simulink model "DT4V_System_Model_v17_ref_speed_R2019a"  (R2023a)
settings: Solver=ode4  StartTime=0.0  StopTime=Config.Tsim  FixedStep=Config.Ts  RelTol=1e-3
undefined symbols (not defined in the file or in its folder): CC, Config, DCL, DiscIntNeverNeededParam, EM, GB, Grid, Inv, LM, Ma_1D, Psw_1D, Rceon_1D, Rec, Vceon_1D
libraries: simulink x3, DT4V_LoadModels x2
(part 1 of 2)
settings Model: TunableVars=Inv,Vceon_1D,Ma_1D,Psw_1D,Rceon_1D  TunableVarsStorageClass=Auto,Auto,Auto,Auto,Auto  TunableVarsTypeQualifier=,,,,  Creator=kjvthuyn  LastModifiedBy=megle
settings SolverCC: AlgebraicLoopSolver=TrustRegion
settings DebuggingCC: UnconnectedInputMsg=warning  UnconnectedOutputMsg=warning  UnconnectedLineMsg=warning
settings ModelReferenceCC: EnableRefExpFcnMdlSchedulingChecks=on
settings SFSimCC: CustomCodeUndefinedFunction=UseInterfaceOnly

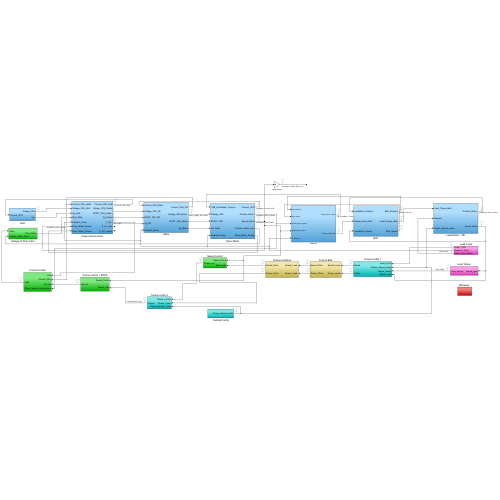
[thumbnail: Simulink's stored preview of the top-level diagram]
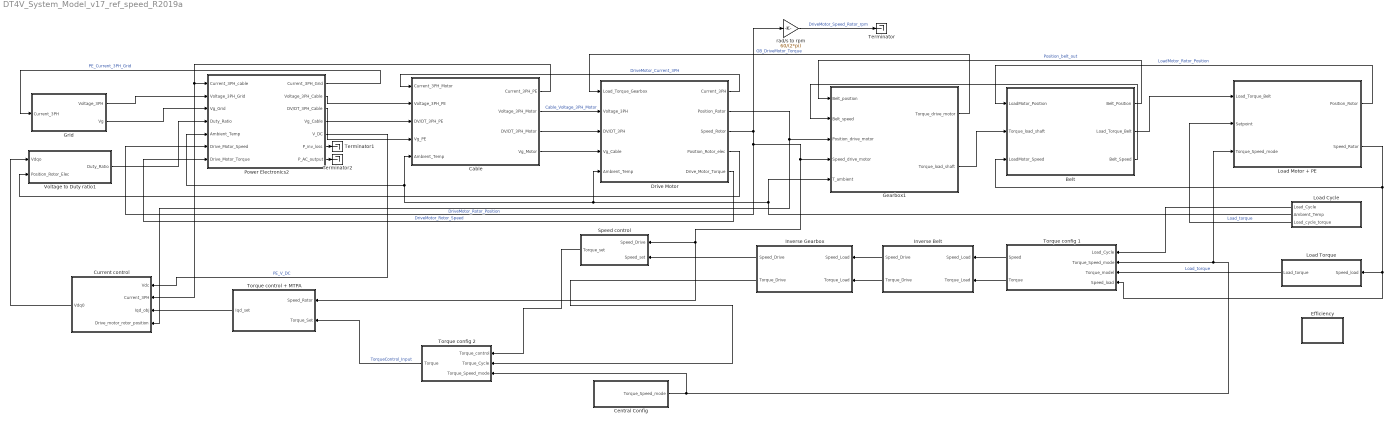
== system DT4V_System_Model_v17_ref_speed_R2019a ==
  Belt : Subsystem
  Cable : Subsystem
  Central Config : Subsystem
  Current control : Subsystem
  Drive Motor : Subsystem
  "Efficiency " : Subsystem
  Gearbox1 : Subsystem
  Grid : Subsystem
  Inverse Belt : Subsystem
  Inverse Gearbox : Subsystem
  Load Cycle : Subsystem
  Load Motor + PE : Subsystem
  Load Torque : Subsystem
  Power Electronics2 : Subsystem
  Speed control : Subsystem
  Terminator : Terminator
  Terminator1 : Terminator
  Terminator2 : Terminator
  Torque config 1 : Subsystem
  Torque config 2 : Subsystem
  Torque control + MTPA : Subsystem
  Voltage to Duty ratio1 : Subsystem
  rad/s to rpm : Gain  Gain=60/(2*pi)
  wires:
  Cable/2("Voltage_3PH_Motor ") -> Drive Motor/2(Voltage_3PH)  "Cable_Voltage_3PH_Motor"
  Cable/3(DV/DT_3PH_Motor) -> Drive Motor/3(DV/DT_3PH)
  Drive Motor/1(Current_3PH) -> Cable/1(Current_3PH_Motor)  "DriveMotor_Current_3PH"
  Power Electronics2/3("DV/DT_3PH_Cable ") -> Cable/3("DV/DT_3PH_PE ")
  Current control/1("Vdq0 ") -> Voltage to Duty ratio1/1(Vdqo)
  Power Electronics2/4(Vg_Cable) -> Cable/4(Vg_PE)
  Cable/4(Vg_Motor) -> Drive Motor/4(Vg_Cable)
  Central Config/1(Torque_Speed_mode) -> Torque config 2/3(Torque_Speed_mode), Torque config 1/2(Torque_Speed_mode), Load Motor + PE/3(Torque_Speed_mode)
  Load Cycle/3(Load_cycle_torque) -> Load Motor + PE/2(Setpoint)  "Load_torque"
  Torque control + MTPA/1(Iqd_set) -> Current control/3(Iqd_obj)
  Inverse Gearbox/2(Torque_Drive) -> Torque config 2/2(Torque_Cycle)
  Speed control/1(Torque_set) -> Torque config 2/1(Torque_control)
  Inverse Gearbox/1(Speed_Drive) -> Speed control/2(Speed_set)
  Load Cycle/2(Ambient_Temp) -> Gearbox1/5(T_ambient), Power Electronics2/5(Ambient_Temp), Cable/5(Ambient_Temp), Drive Motor/5(Ambient_Temp)
  Drive Motor/4(Position_Rotor_elec) -> Voltage to Duty ratio1/2("Position_Rotor_Elec ")
  Voltage to Duty ratio1/1("Duty_Ratio ") -> Power Electronics2/4(Duty_Ratio)
  Power Electronics2/1(Current_3PH_Grid) -> Grid/1(Current_3PH)  "PE_Current_3PH_Grid"
  Grid/2("Vg ") -> Power Electronics2/3("Vg_Grid ")
  Grid/1(Voltage_3PH) -> Power Electronics2/2("Voltage_3PH_Grid ")
  Cable/1(Current_3PH_PE) -> Current control/2(Current_3PH), Power Electronics2/1(Current_3PH_cable)
  Power Electronics2/5("V_DC ") -> Current control/1(Vdc)  "PE_V_DC"
  Drive Motor/2("Position_Rotor ") -> Gearbox1/3(Position_drive_motor), Current control/4(Drive_motor_rotor_position)  "DriveMotor_Rotor_Position"
  Drive Motor/3(Speed_Rotor) -> Power Electronics2/6(Drive_Motor_Speed), Gearbox1/4(Speed_drive_motor), Torque control + MTPA/1(Speed_Rotor), Speed control/1(Speed_Drive), rad/s to rpm/1  "DriveMotor_Rotor_Speed"
  Power Electronics2/2(Voltage_3PH_Cable) -> Cable/2(Voltage_3PH_PE)
  Torque config 2/1(Torque) -> Torque control + MTPA/2(Torque_Set)  "TorqueControl_Input"
  Load Cycle/1(Load_Cycle) -> Torque config 1/1(Load_Cycle)
  rad/s to rpm/1 -> Terminator/1  "DriveMotor_Speed_Rotor_rpm"
  Inverse Belt/1(Speed_Drive) -> Inverse Gearbox/1("Speed_Load ")
  Inverse Belt/2(Torque_Drive) -> Inverse Gearbox/2("Torque_Load ")
  Torque config 1/2(Torque) -> Inverse Belt/2("Torque_Load ")
  Torque config 1/1(Speed) -> Inverse Belt/1("Speed_Load ")
  Belt/2(Load_Torque_Belt) -> Load Motor + PE/1(Load_Torque_Belt)
  Load Motor + PE/1("Position_Rotor ") -> Belt/1(LoadMotor_Position)  "LoadMotor_Rotor_Position"
  Belt/1(Belt_Position) -> Gearbox1/1(Belt_position)  "Position_belt_out"
  Load Motor + PE/2(Speed_Rotor) -> Belt/3(LoadMotor_Speed), Torque config 1/4(Speed_load), Load Torque/1(Speed_load)
  Belt/3(Belt_Speed) -> Gearbox1/2(Belt_speed)
  Power Electronics2/7(P_AC_output) -> Terminator2/1
  Power Electronics2/6(P_inv_loss) -> Terminator1/1
  Gearbox1/1(Torque_drive_motor) -> Drive Motor/1(Load_Torque_Gearbox)  "GB_DriveMotor_Torque"
  Gearbox1/2(Torque_load_shaft) -> Belt/2(Torque_load_shaft)
  Drive Motor/5(Drive_Motor_Torque) -> Power Electronics2/7(Drive_Motor_Torque)
  Load Torque/1(Load_torque) -> Torque config 1/3(Torque_model)  "Load_torque"

== system DT4V_System_Model_v17_ref_speed_R2019a/Belt ==
  note: Ideal belt, no dynamic
  LoadMotor_Position : Inport
  Torque_load_shaft : Inport  Port=2
  LoadMotor_Speed : Inport  Port=3
  position_belt_coef : Gain  Gain=1/3
  speed_belt_coef : Gain  Gain=1/3
  torque_belt_coef : Gain  Gain=1/3
  Belt_Position : Outport
  Load_Torque_Belt : Outport  Port=2
  Belt_Speed : Outport  Port=3
  wires:
  LoadMotor_Speed/1 -> speed_belt_coef/1
  LoadMotor_Position/1 -> position_belt_coef/1
  Torque_load_shaft/1 -> torque_belt_coef/1
  torque_belt_coef/1 -> Load_Torque_Belt/1
  speed_belt_coef/1 -> Belt_Speed/1
  position_belt_coef/1 -> Belt_Position/1

== system DT4V_System_Model_v17_ref_speed_R2019a/Cable ==
  note: Ideal cable, no dynamic
  Current_3PH_Motor : Inport
  Voltage_3PH_PE : Inport  Port=2
  "DV/DT_3PH_PE " : Inport  Port=3
  Vg_PE : Inport  Port=4
  Ambient_Temp : Inport  Port=5
  Current_3PH_PE : Outport
  "Voltage_3PH_Motor " : Outport  Port=2
  DV/DT_3PH_Motor : Outport  Port=3
  Vg_Motor : Outport  Port=4
  wires:
  "DV/DT_3PH_PE "/1 -> DV/DT_3PH_Motor/1
  Vg_PE/1 -> Vg_Motor/1
  Voltage_3PH_PE/1 -> "Voltage_3PH_Motor "/1
  Current_3PH_Motor/1 -> Current_3PH_PE/1

== system DT4V_System_Model_v17_ref_speed_R2019a/Central Config ==
  Constant : Constant  Value=Config.TSm
  Torque_Speed_mode : Outport
  wires:
  Constant/1 -> Torque_Speed_mode/1

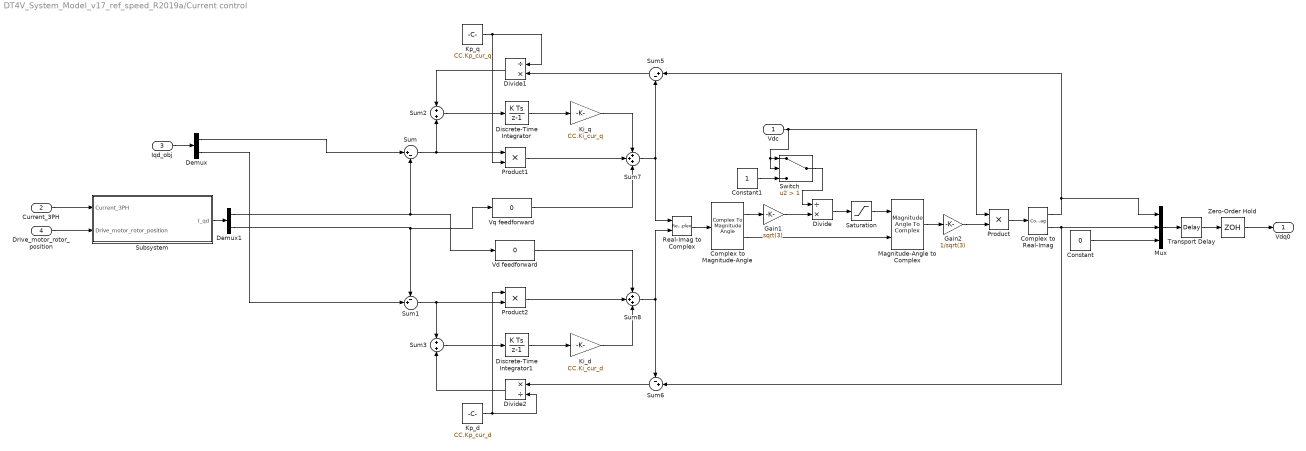
== system DT4V_System_Model_v17_ref_speed_R2019a/Current control ==
  Vdc : Inport
  Current_3PH : Inport  Port=2
  Iqd_obj : Inport  Port=3
  Drive_motor_rotor_position : Inport  Port=4
  Complex to Magnitude-Angle : ComplexToMagnitudeAngle
  Complex to Real-Imag : ComplexToRealImag
  Constant : Constant  Value=0
  Constant1 : Constant
  Demux : Demux  Outputs=2
  Demux1 : Demux  Outputs=2
  Discrete-Time Integrator : DiscreteIntegrator  SampleTime=CC.Ts  ICPrevOutput=DiscIntNeverNeededParam  ICPrevScaledInput=DiscIntNeverNeededParam
  Discrete-Time Integrator1 : DiscreteIntegrator  SampleTime=CC.Ts  ICPrevOutput=DiscIntNeverNeededParam  ICPrevScaledInput=DiscIntNeverNeededParam
  Divide : Product  Inputs=/*
  Divide1 : Product  Inputs=/*
  Divide2 : Product  Inputs=*/
  Gain1 : Gain  Gain=sqrt(3)
  Gain2 : Gain  Gain=1/sqrt(3)
  Ki_d : Gain  Gain=CC.Ki_cur_d
  Ki_q : Gain  Gain=CC.Ki_cur_q
  Kp_d : Constant  Value=CC.Kp_cur_d
  Kp_q : Constant  Value=CC.Kp_cur_q
  Magnitude-Angle to Complex : MagnitudeAngleToComplex
  Mux : Mux  Inputs=3
  Product : Product
  Product1 : Product
  Product2 : Product
  Real-Imag to Complex : RealImagToComplex
  Saturation : Saturate  UpperLimit=2  LowerLimit=0  LinearizeAsGain=off
  Subsystem : Subsystem
  Sum : Sum  Inputs=|+-
  Sum1 : Sum  Inputs=-+|
  Sum2 : Sum  Inputs=+|+
  Sum3 : Sum  Inputs=+|+
  Sum5 : Sum  Inputs=|+-
  Sum6 : Sum  Inputs=-+|
  Sum7 : Sum  Inputs=+++
  Sum8 : Sum  Inputs=+++
  Switch : Switch  Criteria=u2 > Threshold  Threshold=1  SaturateOnIntegerOverflow=off  InputSameDT=off
  Transport Delay : TransportDelay  DelayTime=CC.Ts/2
  Vd feedforward : Fcn  Expr=0
  Vq feedforward : Fcn  Expr=0
  Zero-Order Hold : ZeroOrderHold  SampleTime=CC.Ts
  "Vdq0 " : Outport
  wires:
  Current_3PH/1 -> Subsystem/1(Current_3PH)
  Drive_motor_rotor_position/1 -> Subsystem/2(Drive_motor_rotor_position)
  Divide2/1 -> Sum3/2
  Vq feedforward/1 -> Sum7/3
  Sum3/1 -> Discrete-Time Integrator1/1
  Sum8/1 -> Sum6/1, Real-Imag to Complex/2
  Ki_q/1 -> Sum7/1
  Sum7/1 -> Sum5/2, Real-Imag to Complex/1
  Divide1/1 -> Sum2/1
  Sum5/1 -> Divide1/2
  Complex to Magnitude-Angle/2 -> Magnitude-Angle to Complex/2
  Gain2/1 -> Product/2
  Divide/1 -> Saturation/1
  Real-Imag to Complex/1 -> Complex to Magnitude-Angle/1
  Discrete-Time Integrator/1 -> Ki_q/1
  Complex to Magnitude-Angle/1 -> Gain1/1
  Product2/1 -> Sum8/2
  Product1/1 -> Sum7/2
  Product/1 -> Complex to Real-Imag/1
  Demux/1 -> Sum/1
  Sum1/1 -> Sum3/1, Product2/2
  Sum/1 -> Sum2/2, Product1/1
  Kp_q/1 -> Divide1/1, Product1/2
  Kp_d/1 -> Divide2/2, Product2/1
  Saturation/1 -> Magnitude-Angle to Complex/1
  Demux/2 -> Sum1/2
  Gain1/1 -> Divide/2
  Demux1/2 -> Sum1/1, Vq feedforward/1
  Complex to Real-Imag/2 -> Mux/2, Sum6/2
  Magnitude-Angle to Complex/1 -> Gain2/1
  Discrete-Time Integrator1/1 -> Ki_d/1
  Demux1/1 -> Sum/2, Vd feedforward/1
  Sum6/1 -> Divide2/1
  Ki_d/1 -> Sum8/3
  Vd feedforward/1 -> Sum8/1
  Sum2/1 -> Discrete-Time Integrator/1
  Iqd_obj/1 -> Demux/1
  Subsystem/1("I_qd ") -> Demux1/1
  Constant/1 -> Mux/3
  Complex to Real-Imag/1 -> Mux/1, Sum5/1
  Constant1/1 -> Switch/3
  Vdc/1 -> Switch/1, Switch/2, Product/1
  Switch/1 -> Divide/1
  Mux/1 -> Transport Delay/1
  Zero-Order Hold/1 -> "Vdq0 "/1
  Transport Delay/1 -> Zero-Order Hold/1

== system DT4V_System_Model_v17_ref_speed_R2019a/Drive Motor ==
  Load_Torque_Gearbox : Inport
  Voltage_3PH : Inport  Port=2
  DV/DT_3PH : Inport  Port=3
  Vg_Cable : Inport  Port=4
  Ambient_Temp : Inport  Port=5
  Electromagnetic Model : Subsystem
  Mechanical model : Subsystem
  Position mech. to elec. : Gain  Gain=EM.Np
  To Workspace1 : ToWorkspace  VariableName=drive_motor_torque  SampleTime=-1
      settings: Save2DSignal=2-D array (concatenate along first dimension)
  To Workspace2 : ToWorkspace  VariableName=drive_motor_current  SampleTime=-1
      settings: Save2DSignal=2-D array (concatenate along first dimension)
  Current_3PH : Outport
  "Position_Rotor " : Outport  Port=2
  Speed_Rotor : Outport  Port=3
  Position_Rotor_elec : Outport  Port=4
  Drive_Motor_Torque : Outport  Port=5
  wires:
  Voltage_3PH/1 -> Electromagnetic Model/1(Voltage_3PH)
  DV/DT_3PH/1 -> Electromagnetic Model/2("DV/DT_3PH ")
  Electromagnetic Model/1("Current_3PH ") -> To Workspace2/1, Current_3PH/1
  Electromagnetic Model/2("EM_Torque ") -> To Workspace1/1, Drive_Motor_Torque/1, Mechanical model/1(EM_Torque)  "DriveMotor_EM_Torque"
  Load_Torque_Gearbox/1 -> Mechanical model/2(Load_Torque)
  Mechanical model/1("Position_Rotor ") -> Electromagnetic Model/4("Position_rotor "), Position mech. to elec./1, "Position_Rotor "/1  "DriveMotor_Rotor_Position"
  Mechanical model/2("Speed_Rotor ") -> Electromagnetic Model/3("Speed_rotor "), Speed_Rotor/1  "DriveMotor_Rotor_Speed"
  Position mech. to elec./1 -> Position_Rotor_elec/1

== system DT4V_System_Model_v17_ref_speed_R2019a/Efficiency  ==
  Abs : Abs  SaturateOnIntegerOverflow=off
  Abs1 : Abs  SaturateOnIntegerOverflow=off
  Divide : Product  Inputs=*/
  To Workspace1 : ToWorkspace  VariableName=efficiency  SampleTime=-1
      settings: Save2DSignal=2-D array (concatenate along first dimension)
  wires:
  [input_power] -> Abs1/1
  [output_power] -> Abs/1
  Divide/1 -> To Workspace1/1
  Abs/1 -> Divide/1
  Abs1/1 -> Divide/2

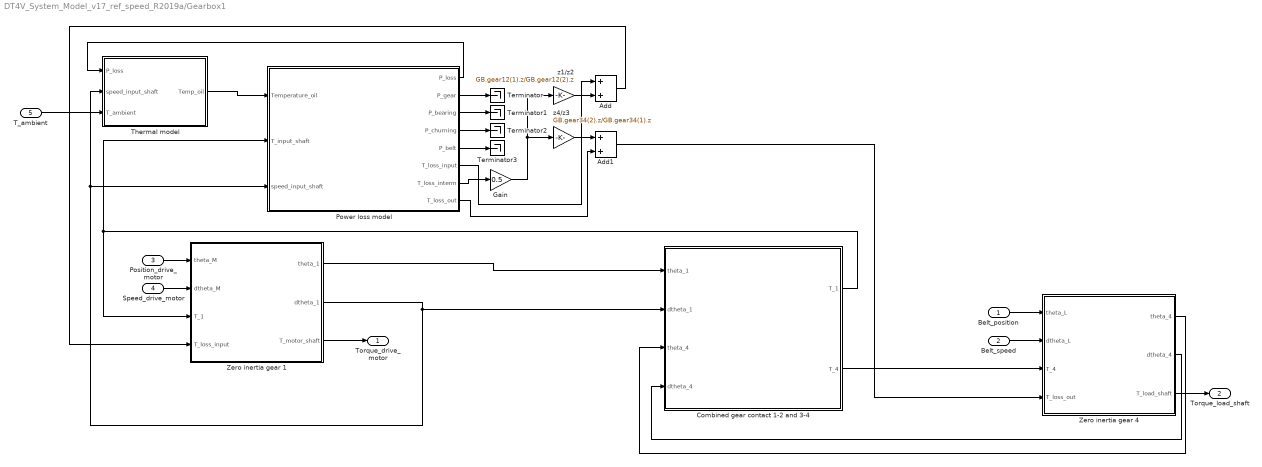
== system DT4V_System_Model_v17_ref_speed_R2019a/Gearbox1 ==
  Belt_position : Inport
  Belt_speed : Inport  Port=2
  Position_drive_motor : Inport  Port=3
  Speed_drive_motor : Inport  Port=4
  T_ambient : Inport  Port=5
  Add : Sum
  Add1 : Sum
  Combined gear contact 1-2 and 3-4 : Subsystem
  Gain : Gain  Gain=0.5
  Power loss model : Subsystem
  Terminator{,1..3} (4 alike) : Terminator
  Thermal model : Subsystem
  Zero inertia gear 1 : Subsystem
  Zero inertia gear 4 : Subsystem
  z1/z2 : Gain  Gain=GB.gear12(1).z/GB.gear12(2).z
  z4/z3 : Gain  Gain=GB.gear34(2).z/GB.gear34(1).z
  Torque_drive_motor : Outport
  Torque_load_shaft : Outport  Port=2
  wires:
  Position_drive_motor/1 -> Zero inertia gear 1/1(theta_M)
  Zero inertia gear 1/3(T_motor_shaft) -> Torque_drive_motor/1
  Speed_drive_motor/1 -> Zero inertia gear 1/2(dtheta_M)
  Zero inertia gear 1/1(theta_1) -> Combined gear contact 1-2 and 3-4/1(theta_1)
  Belt_position/1 -> Zero inertia gear 4/1(theta_L)
  Belt_speed/1 -> Zero inertia gear 4/2(dtheta_L)
  Zero inertia gear 4/3(T_load_shaft) -> Torque_load_shaft/1
  Power loss model/4(P_churning) -> Terminator2/1
  Power loss model/3(P_bearing) -> Terminator1/1
  Power loss model/2(P_gear) -> Terminator/1
  Power loss model/6(T_loss_input) -> Add/1
  Power loss model/8(T_loss_out) -> Add1/2
  Power loss model/1(P_loss) -> Thermal model/1(P_loss)
  Thermal model/1(Temp_oil) -> Power loss model/1(Temperature_oil)
  Zero inertia gear 1/2(dtheta_1) -> Thermal model/2(speed_input_shaft), Power loss model/3(speed_input_shaft), Combined gear contact 1-2 and 3-4/2(dtheta_1)
  Combined gear contact 1-2 and 3-4/1(T_1) -> Zero inertia gear 1/3(T_1), Power loss model/2(T_input_shaft)
  T_ambient/1 -> Thermal model/3(T_ambient)
  Zero inertia gear 4/1(theta_4) -> Combined gear contact 1-2 and 3-4/3(theta_4)
  Zero inertia gear 4/2(dtheta_4) -> Combined gear contact 1-2 and 3-4/4(dtheta_4)
  Combined gear contact 1-2 and 3-4/2(T_4) -> Zero inertia gear 4/3(T_4)
  Power loss model/7(T_loss_interm) -> Gain/1
  Gain/1 -> z4/z3/1, z1/z2/1
  z1/z2/1 -> Add/2
  Add/1 -> Zero inertia gear 1/4(T_loss_input)
  z4/z3/1 -> Add1/1
  Power loss model/5(P_belt) -> Terminator3/1
  Add1/1 -> Zero inertia gear 4/4(T_loss_out)

== system DT4V_System_Model_v17_ref_speed_R2019a/Grid ==
  Current_3PH : Inport
  Constant : Constant  Value=0
  Mux1 : Mux  Inputs=3
  Sine Wave A : Sin  Amplitude=Grid.vol.Vph_C_v  Frequency=50*2*pi  SampleTime=0
  Sine Wave B : Sin  Amplitude=Grid.vol.Vph_C_v  Frequency=50*2*pi  Phase=-2*pi/3  SampleTime=0
  Sine Wave C : Sin  Amplitude=Grid.vol.Vph_C_v  Frequency=50*2*pi  Phase=2*pi/3  SampleTime=0
  Terminator : Terminator
  Voltage_3PH : Outport
  "Vg " : Outport  Port=2
  wires:
  Current_3PH/1 -> Terminator/1
  Constant/1 -> "Vg "/1
  Sine Wave C/1 -> Mux1/3
  Sine Wave B/1 -> Mux1/2
  Sine Wave A/1 -> Mux1/1
  Mux1/1 -> Voltage_3PH/1

== system DT4V_System_Model_v17_ref_speed_R2019a/Inverse Belt ==
  "Speed_Load " : Inport
  "Torque_Load " : Inport  Port=2
  Multiply : Gain  Gain=3
  Multiply1 : Gain  Gain=1/3
  Speed_Drive : Outport
  Torque_Drive : Outport  Port=2
  wires:
  Multiply/1 -> Torque_Drive/1
  "Torque_Load "/1 -> Multiply/1
  Multiply1/1 -> Speed_Drive/1
  "Speed_Load "/1 -> Multiply1/1

== system DT4V_System_Model_v17_ref_speed_R2019a/Inverse Gearbox ==
  "Speed_Load " : Inport
  "Torque_Load " : Inport  Port=2
  Multiply : Gain  Gain=GB.gear12(1).z/GB.gear12(2).z*GB.gear34(1).z/GB.gear34(2).z
  Multiply1 : Gain  Gain=GB.gear12(2).z/GB.gear12(1).z*GB.gear34(2).z/GB.gear34(1).z
  Speed_Drive : Outport
  Torque_Drive : Outport  Port=2
  wires:
  "Speed_Load "/1 -> Multiply1/1
  Multiply1/1 -> Speed_Drive/1
  "Torque_Load "/1 -> Multiply/1
  Multiply/1 -> Torque_Drive/1

== system DT4V_System_Model_v17_ref_speed_R2019a/Load Cycle ==
  Add : Sum
  Constant1 : Constant  Value=25
  Constant2 : Constant  Value=0.1
  From Workspace1 : FromWorkspace  VariableName=speed_input
  Load cycle : Subsystem
  Product : Product
  To Workspace1 : ToWorkspace  VariableName=output_power1  SampleTime=-1
      settings: Save2DSignal=2-D array (concatenate along first dimension)
  reverse power flow : Gain  Gain=-1
  Load_Cycle : Outport
  Ambient_Temp : Outport  Port=2
  Load_cycle_torque : Outport  Port=3
  tag scope: output_power=global
  wires:
  Constant1/1 -> Ambient_Temp/1
  reverse power flow/1 -> Load_cycle_torque/1
  Constant2/1 -> Add/1
  Product/1 -> [output_power], To Workspace1/1
  From Workspace1/1 -> Add/2
  Load cycle/1(Torque_Load) -> Product/2, reverse power flow/1
  Add/1 -> Load cycle/1(Speed_load), Product/1, Load_Cycle/1

== system DT4V_System_Model_v17_ref_speed_R2019a/Load Motor + PE ==
  Load_Torque_Belt : Inport
  Setpoint : Inport  Port=2
  Torque_Speed_mode : Inport  Port=3
  Constant : Constant  Value=0
  Integrator3 : Integrator
  Mechanical model : Subsystem
  Switch{,1..3} (4 alike) : Switch  Criteria=u2 > Threshold  Threshold=0.5  SaturateOnIntegerOverflow=off  InputSameDT=off
  "Position_Rotor " : Outport
  Speed_Rotor : Outport  Port=2
  wires:
  Integrator3/1 -> Switch3/1
  Switch/1 -> Switch2/1, Integrator3/1
  Setpoint/1 -> Switch1/3, Switch/1
  Constant/1 -> Switch/3, Switch1/1
  Torque_Speed_mode/1 -> Switch/2, Switch3/2, Switch2/2, Switch1/2
  Switch2/1 -> Speed_Rotor/1
  Switch1/1 -> Mechanical model/1(EM_Torque)
  Load_Torque_Belt/1 -> Mechanical model/2(Load_Torque)
  Mechanical model/1("Position_Rotor ") -> Switch3/3  "LoadMotor_Rotor_Position"
  Switch3/1 -> "Position_Rotor "/1
  Mechanical model/2("Speed_Rotor ") -> Switch2/3  "LoadMotor_Rotor_Speed"

== system DT4V_System_Model_v17_ref_speed_R2019a/Load Torque ==
  Speed_load : Inport
  Load cycle : Subsystem
  reverse power flow : Gain  Gain=-1
  Load_torque : Outport
  wires:
  reverse power flow/1 -> Load_torque/1
  Load cycle/1(Torque_Load) -> reverse power flow/1
  Speed_load/1 -> Load cycle/1(Speed_load)

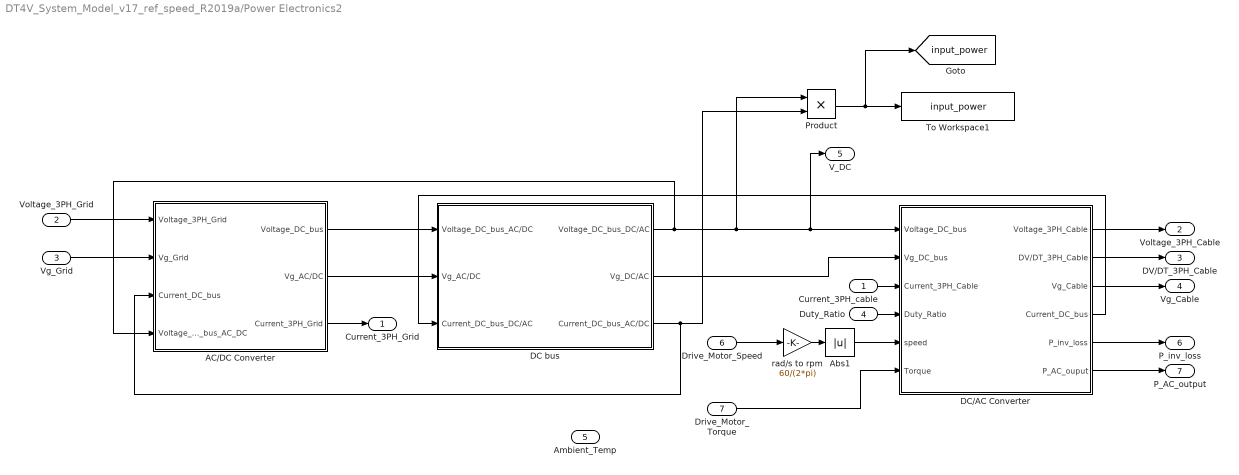
== system DT4V_System_Model_v17_ref_speed_R2019a/Power Electronics2 ==
  Current_3PH_cable : Inport
  "Voltage_3PH_Grid " : Inport  Port=2
  "Vg_Grid " : Inport  Port=3
  Duty_Ratio : Inport  Port=4
  Ambient_Temp : Inport  Port=5
  Drive_Motor_Speed : Inport  Port=6
  Drive_Motor_Torque : Inport  Port=7
  AC/DC Converter : Subsystem
  Abs1 : Abs  SaturateOnIntegerOverflow=off
  "DC bus " : Subsystem
  DC/AC Converter : Subsystem
  Product : Product
  To Workspace1 : ToWorkspace  VariableName=input_power  SampleTime=-1
      settings: Save2DSignal=2-D array (concatenate along first dimension)
  rad/s to rpm : Gain  Gain=60/(2*pi)
  Current_3PH_Grid : Outport
  Voltage_3PH_Cable : Outport  Port=2
  "DV/DT_3PH_Cable " : Outport  Port=3
  Vg_Cable : Outport  Port=4
  "V_DC " : Outport  Port=5
  P_inv_loss : Outport  Port=6
  P_AC_output : Outport  Port=7
  tag scope: input_power=global
  wires:
  DC/AC Converter/4(Current_DC_bus) -> "DC bus "/3(Current_DC_bus_DC/AC)
  Current_3PH_cable/1 -> DC/AC Converter/3("Current_3PH_Cable ")
  "Vg_Grid "/1 -> AC/DC Converter/2("Vg_Grid ")
  AC/DC Converter/1(Voltage_DC_bus) -> "DC bus "/1(Voltage_DC_bus_AC/DC)
  "DC bus "/3(Current_DC_bus_AC/DC) -> Product/2, AC/DC Converter/3(Current_DC_bus)
  DC/AC Converter/1(Voltage_3PH_Cable) -> Voltage_3PH_Cable/1
  DC/AC Converter/3("Vg_Cable ") -> Vg_Cable/1
  "Voltage_3PH_Grid "/1 -> AC/DC Converter/1(Voltage_3PH_Grid)
  Duty_Ratio/1 -> DC/AC Converter/4(Duty_Ratio)
  AC/DC Converter/3(Current_3PH_Grid) -> Current_3PH_Grid/1
  AC/DC Converter/2(Vg_AC/DC) -> "DC bus "/2(Vg_AC/DC)
  DC/AC Converter/2(DV/DT_3PH_Cable) -> "DV/DT_3PH_Cable "/1
  DC/AC Converter/6(P_AC_ouput) -> P_AC_output/1
  DC/AC Converter/5(P_inv_loss) -> P_inv_loss/1
  Drive_Motor_Speed/1 -> rad/s to rpm/1
  rad/s to rpm/1 -> Abs1/1
  Product/1 -> [input_power], To Workspace1/1
  "DC bus "/1(Voltage_DC_bus_DC/AC) -> AC/DC Converter/4(Voltage_DC_bus_AC_DC), Product/1, "V_DC "/1, DC/AC Converter/1(Voltage_DC_bus)
  "DC bus "/2(Vg_DC/AC) -> DC/AC Converter/2(Vg_DC_bus)
  Drive_Motor_Torque/1 -> DC/AC Converter/6(Torque)
  Abs1/1 -> DC/AC Converter/5(speed)

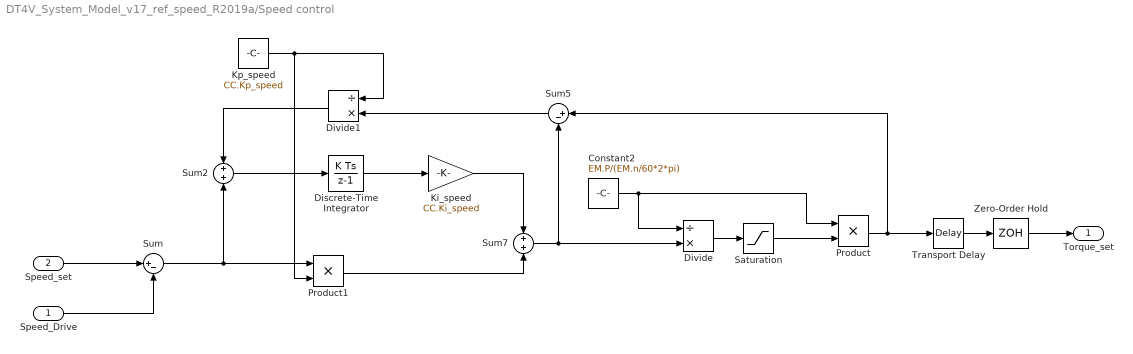
== system DT4V_System_Model_v17_ref_speed_R2019a/Speed control ==
  Speed_Drive : Inport
  Speed_set : Inport  Port=2
  Constant2 : Constant  Value=EM.P/(EM.n/60*2*pi)
  Discrete-Time Integrator : DiscreteIntegrator  SampleTime=CC.Ts_speed  ICPrevOutput=DiscIntNeverNeededParam  ICPrevScaledInput=DiscIntNeverNeededParam
  Divide : Product  Inputs=/*
  Divide1 : Product  Inputs=/*
  Ki_speed : Gain  Gain=CC.Ki_speed
  "Kp_speed " : Constant  Value=CC.Kp_speed
  Product : Product
  Product1 : Product
  Saturation : Saturate  UpperLimit=1  LowerLimit=-1  LinearizeAsGain=off
  Sum : Sum  Inputs=|+-
  Sum2 : Sum  Inputs=+|+
  Sum5 : Sum  Inputs=|+-
  Sum7 : Sum
  Transport Delay : TransportDelay  DelayTime=CC.Ts_speed/2
  Zero-Order Hold : ZeroOrderHold  SampleTime=CC.Ts_speed
  Torque_set : Outport
  wires:
  Sum7/1 -> Divide/2, Sum5/2
  Sum/1 -> Sum2/2, Product1/1
  Discrete-Time Integrator/1 -> Ki_speed/1
  Sum5/1 -> Divide1/2
  Constant2/1 -> Divide/1, Product/1
  Sum2/1 -> Discrete-Time Integrator/1
  Speed_Drive/1 -> Sum/2
  "Kp_speed "/1 -> Divide1/1, Product1/2
  Speed_set/1 -> Sum/1
  Saturation/1 -> Product/2
  Ki_speed/1 -> Sum7/1
  Divide/1 -> Saturation/1
  Divide1/1 -> Sum2/1
  Product1/1 -> Sum7/2
  Product/1 -> Transport Delay/1, Sum5/1
  Transport Delay/1 -> Zero-Order Hold/1
  Zero-Order Hold/1 -> Torque_set/1

== system DT4V_System_Model_v17_ref_speed_R2019a/Torque config 1 ==
  Load_Cycle : Inport
  Torque_Speed_mode : Inport  Port=2
  Torque_model : Inport  Port=3
  Speed_load : Inport  Port=4
  Switch : Switch  Criteria=u2 > Threshold  Threshold=0.5  SaturateOnIntegerOverflow=off  InputSameDT=off
  Switch1 : Switch  Criteria=u2 > Threshold  Threshold=0.5  SaturateOnIntegerOverflow=off  InputSameDT=off
  Speed : Outport
  Torque : Outport  Port=2
  wires:
  Torque_model/1 -> Switch/1
  Torque_Speed_mode/1 -> Switch/2, Switch1/2
  Load_Cycle/1 -> Switch/3, Switch1/3
  Speed_load/1 -> Switch1/1
  Switch1/1 -> Speed/1
  Switch/1 -> Torque/1

== system DT4V_System_Model_v17_ref_speed_R2019a/Torque config 2 ==
  Torque_control : Inport
  Torque_Cycle : Inport  Port=2
  Torque_Speed_mode : Inport  Port=3
  Switch : Switch  Criteria=u2 > Threshold  Threshold=0.5  SaturateOnIntegerOverflow=off  InputSameDT=off
  Torque : Outport
  wires:
  Switch/1 -> Torque/1
  Torque_Speed_mode/1 -> Switch/2
  Torque_Cycle/1 -> Switch/1
  Torque_control/1 -> Switch/3

== system DT4V_System_Model_v17_ref_speed_R2019a/Torque control + MTPA ==
  note: Torque -> current setpoint Open loop
      | as no Torque measurement foreseen in practice
      | No MTPA
  Speed_Rotor : Inport
  Torque_Set : Inport  Port=2
  Gain1 : Gain  Gain=1/(-3/2*EM.Np*EM.L_d*EM.i_mag)
  "Id_ref " : Constant  Value=0
  Mux : Mux  Inputs=2
  Iqd_set : Outport
  wires:
  Mux/1 -> Iqd_set/1
  "Id_ref "/1 -> Mux/2
  Torque_Set/1 -> Gain1/1
  Gain1/1 -> Mux/1

== system DT4V_System_Model_v17_ref_speed_R2019a/Voltage to Duty ratio1 ==
  note: The a -axis and the d -axis are initially aligned.
      | The q-axis is leading the d-axis
      | Not power invariant transforamation
  Vdqo : Inport
  "Position_Rotor_Elec " : Inport  Port=2
  Gate signal generator : Subsystem
  Saturation : Saturate  UpperLimit=DCL.Cap.Vdc_C_v/2  LowerLimit=-DCL.Cap.Vdc_C_v/2
  dqo_to_abc : Subsystem
  "Duty_Ratio " : Outport
  wires:
  dqo_to_abc/1(abc) -> Saturation/1
  "Position_Rotor_Elec "/1 -> dqo_to_abc/2(theta)
  Saturation/1 -> Gate signal generator/1(In1)
  Vdqo/1 -> dqo_to_abc/1("Vdqo ")
  Gate signal generator/1(Out1) -> "Duty_Ratio "/1

== system DT4V_System_Model_v17_ref_speed_R2019a/Current control/Subsystem ==
  Current_3PH : Inport
  Drive_motor_rotor_position : Inport  Port=2
  Constant : Constant  Value=EM.Np
  Demux : Demux  Outputs=2
      settings: DisplayOption=none
  Mux : Mux  Inputs=2
  Product{,1,3..4,7} (5 alike) : Product  InputSameDT=on  SaturateOnIntegerOverflow=on  OutDataTypeStr=Inherit: Same as first input
  Sum1 : Sum  Inputs=|++  InputSameDT=on  SaturateOnIntegerOverflow=on  OutDataTypeStr=Inherit: Same as first input
  Sum4 : Sum  Inputs=|+-  InputSameDT=on  SaturateOnIntegerOverflow=on  OutDataTypeStr=Inherit: Same as first input
  Tclark : Gain  Gain=EM.TaA  Multiplication=Matrix(K*u)  SaturateOnIntegerOverflow=on  OutDataTypeStr=Inherit: Same as input  ParamDataTypeStr=Inherit: Same as input
  Trigonometric Function2 : Trigonometry  Operator=cos
  Trigonometric Function3 : Trigonometry
  "I_qd " : Outport
  wires:
  Drive_motor_rotor_position/1 -> Product/1
  Trigonometric Function3/1 -> Product4/2, Product7/2
  Product/1 -> Trigonometric Function2/1, Trigonometric Function3/1
  Constant/1 -> Product/2
  Tclark/1 -> Demux/1
  Demux/1 -> Product1/1, Product7/1
  Trigonometric Function2/1 -> Product1/2, Product3/2
  Sum4/1 -> Mux/2
  Sum1/1 -> Mux/1
  Product7/1 -> Sum4/2
  Product4/1 -> Sum1/2
  Current_3PH/1 -> Tclark/1
  Product1/1 -> Sum1/1
  Demux/2 -> Product3/1, Product4/1
  Product3/1 -> Sum4/1
  Mux/1 -> "I_qd "/1

== system DT4V_System_Model_v17_ref_speed_R2019a/Drive Motor/Electromagnetic Model ==
  Voltage_3PH : Inport
  "DV/DT_3PH " : Inport  Port=2
  "Speed_rotor " : Inport  Port=3
  "Position_rotor " : Inport  Port=4
  Constant input voltage : Constant  Value=400
  "DQ-transform " : Subsystem
  Electromagnetic model : Subsystem
  Inverse DQ-transform : Subsystem
  Loss model : Subsystem
  Manual Switch : ManualSwitch  CurrentSetting=0
  Terminator : Terminator
  Terminator1 : Terminator
  "Current_3PH " : Outport
  "EM_Torque " : Outport  Port=2
  wires:
  Electromagnetic model/2("i_d ") -> Inverse DQ-transform/2(i_d)
  "DQ-transform "/1(V_q) -> Electromagnetic model/1("V_q ")
  Electromagnetic model/1("i_q ") -> Loss model/1(Current_q_axis), Inverse DQ-transform/1(i_q)
  Voltage_3PH/1 -> "DQ-transform "/1(Voltage_3PH)
  Inverse DQ-transform/1(Current_3PH) -> "Current_3PH "/1
  "Speed_rotor "/1 -> Electromagnetic model/3("omega_mech ")
  "Position_rotor "/1 -> Inverse DQ-transform/3(Rotor_position), "DQ-transform "/2(Rotor_position)
  Manual Switch/1 -> Electromagnetic model/2("V_d ")
  "DQ-transform "/2("V_d ") -> Manual Switch/2
  Constant input voltage/1 -> Manual Switch/1
  Loss model/1("Copper Loss ") -> Terminator/1  "DriveMotor_LossCopper"
  Electromagnetic model/3("T_em ") -> Loss model/2(EM Torque)
  Electromagnetic model/4(omega_mech) -> Loss model/3(Rotor speed)
  Loss model/3(T_mec) -> "EM_Torque "/1
  Loss model/2(Iron Loss) -> Terminator1/1

== system DT4V_System_Model_v17_ref_speed_R2019a/Drive Motor/Mechanical model ==
  EM_Torque : Inport
  Load_Torque : Inport  Port=2
  Integrator1 : Integrator  ZeroCross=off
  Integrator3 : Integrator
  Multiply : Gain  Gain=1/EM.J
  Sum : Sum
  Sum2 : Sum  Inputs=|++
  bias speed : Constant  Value=0.00005
  "Position_Rotor " : Outport
  "Speed_Rotor " : Outport  Port=2
  wires:
  Integrator3/1 -> "Position_Rotor "/1
  EM_Torque/1 -> Sum/1
  Sum2/1 -> Integrator3/1, "Speed_Rotor "/1
  Integrator1/1 -> Sum2/1
  Load_Torque/1 -> Sum/2
  Multiply/1 -> Integrator1/1
  bias speed/1 -> Sum2/2
  Sum/1 -> Multiply/1

== system DT4V_System_Model_v17_ref_speed_R2019a/Gearbox1/Combined gear contact 1-2 and 3-4 ==
  theta_1 : Inport
  dtheta_1 : Inport  Port=2
  theta_4 : Inport  Port=3
  dtheta_4 : Inport  Port=4
  "Combined contact 1-2, 3-4" : Subsystem
  Constant : Constant  Value=GB.gear34(1).R
  Constant1 : Constant  Value=GB.gear12(1).R
  Constant2 : Constant  Value=GB.gear12(2).R
  Constant3 : Constant  Value=GB.pair12.c_mesh
  Constant4 : Constant  Value=GB.pair12.k_mesh
  Constant5 : Constant  Value=GB.gear34(2).R
  Constant6 : Constant  Value=GB.pair34.k_mesh
  Constant7 : Constant  Value=GB.pair34.c_mesh
  T_1 : Outport
  T_4 : Outport  Port=2
  wires:
  "Combined contact 1-2, 3-4"/1(T_1) -> T_1/1
  "Combined contact 1-2, 3-4"/2(T_4) -> T_4/1
  dtheta_1/1 -> "Combined contact 1-2, 3-4"/2(dtheta1)
  Constant1/1 -> "Combined contact 1-2, 3-4"/5(R1)
  Constant2/1 -> "Combined contact 1-2, 3-4"/6(R2)
  Constant3/1 -> "Combined contact 1-2, 3-4"/11(c_mesh_12)
  theta_1/1 -> "Combined contact 1-2, 3-4"/1(theta1)
  Constant4/1 -> "Combined contact 1-2, 3-4"/9(k_mesh_12)
  Constant/1 -> "Combined contact 1-2, 3-4"/7(R3)
  Constant5/1 -> "Combined contact 1-2, 3-4"/8(R4)
  Constant6/1 -> "Combined contact 1-2, 3-4"/10(k_mesh_34)
  Constant7/1 -> "Combined contact 1-2, 3-4"/12(c_mesh_34)
  theta_4/1 -> "Combined contact 1-2, 3-4"/3(theta4)
  dtheta_4/1 -> "Combined contact 1-2, 3-4"/4(dtheta4)

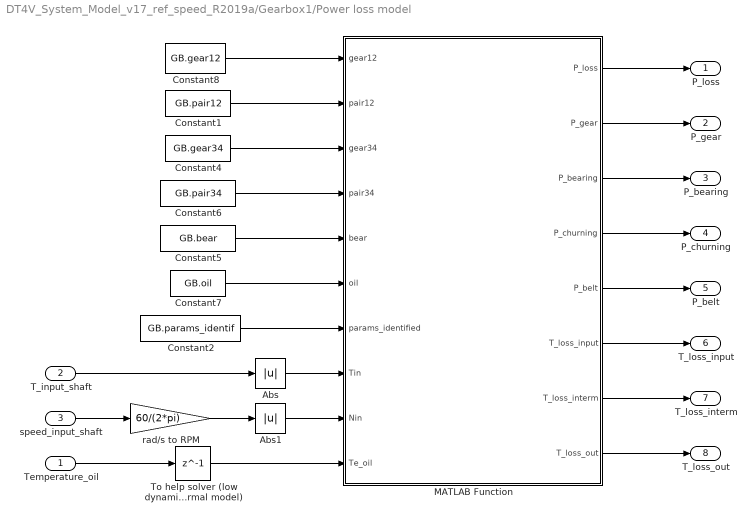
== system DT4V_System_Model_v17_ref_speed_R2019a/Gearbox1/Power loss model ==
  Temperature_oil : Inport
  T_input_shaft : Inport  Port=2
  speed_input_shaft : Inport  Port=3
  Abs : Abs  SaturateOnIntegerOverflow=off
  Abs1 : Abs  SaturateOnIntegerOverflow=off
  Constant1 : Constant  Value=GB.pair12  OutDataTypeStr=Bus: pair12
  Constant2 : Constant  Value=GB.params_identif  OutDataTypeStr=Bus: params_identif
  Constant4 : Constant  Value=GB.gear34  OutDataTypeStr=Bus: gear34
  Constant5 : Constant  Value=GB.bear  OutDataTypeStr=Bus: bear
  Constant6 : Constant  Value=GB.pair34  OutDataTypeStr=Bus: pair34
  Constant7 : Constant  Value=GB.oil  OutDataTypeStr=Bus: oil
  Constant8 : Constant  Value=GB.gear12  OutDataTypeStr=Bus: gear12
  MATLAB Function : MATLAB Function  TreatAsAtomicUnit=on
  To help solver (low dynamics thermal model) : Delay  DelayLength=1  InitialCondition=0
  rad/s to RPM : Gain  Gain=60/(2*pi)
  P_loss : Outport  OutDataTypeStr=double
  P_gear : Outport  Port=2  OutDataTypeStr=double
  P_bearing : Outport  Port=3  OutDataTypeStr=double
  P_churning : Outport  Port=4  OutDataTypeStr=double
  P_belt : Outport  Port=5  OutDataTypeStr=double
  T_loss_input : Outport  Port=6  OutDataTypeStr=double
  T_loss_interm : Outport  Port=7  OutDataTypeStr=double
  T_loss_out : Outport  Port=8  OutDataTypeStr=double
  wires:
  Constant5/1 -> MATLAB Function/5(bear)
  T_input_shaft/1 -> Abs/1
  MATLAB Function/3(P_bearing) -> P_bearing/1
  MATLAB Function/2(P_gear) -> P_gear/1
  Constant4/1 -> MATLAB Function/3(gear34)
  Constant6/1 -> MATLAB Function/4(pair34)
  Constant7/1 -> MATLAB Function/6(oil)
  Constant1/1 -> MATLAB Function/2(pair12)
  Constant8/1 -> MATLAB Function/1(gear12)
  speed_input_shaft/1 -> rad/s to RPM/1
  MATLAB Function/4(P_churning) -> P_churning/1
  MATLAB Function/1(P_loss) -> P_loss/1
  MATLAB Function/6(T_loss_input) -> T_loss_input/1
  MATLAB Function/7(T_loss_interm) -> T_loss_interm/1
  MATLAB Function/8(T_loss_out) -> T_loss_out/1
  rad/s to RPM/1 -> Abs1/1
  Abs/1 -> MATLAB Function/8(Tin)
  Abs1/1 -> MATLAB Function/9(Nin)
  Temperature_oil/1 -> To help solver (low dynamics thermal model)/1
  To help solver (low dynamics thermal model)/1 -> MATLAB Function/10(Te_oil)
  Constant2/1 -> MATLAB Function/7(params_identified)
  MATLAB Function/5(P_belt) -> P_belt/1

== system DT4V_System_Model_v17_ref_speed_R2019a/Gearbox1/Thermal model ==
  P_loss : Inport
  speed_input_shaft : Inport  Port=2
  T_ambient : Inport  Port=3
  Abs : Abs  SaturateOnIntegerOverflow=off
  Heat equation : Subsystem
  MATLAB Function : MATLAB Function  TreatAsAtomicUnit=on
  Temp_oil : Outport
  wires:
  P_loss/1 -> Heat equation/1(P_loss)
  Heat equation/1(T) -> MATLAB Function/2(TSump), Temp_oil/1
  T_ambient/1 -> MATLAB Function/3(TAmb), Heat equation/3(T_ambient)
  speed_input_shaft/1 -> MATLAB Function/1(w)
  MATLAB Function/1(hAEq) -> Abs/1
  Abs/1 -> Heat equation/2(UA)

== system DT4V_System_Model_v17_ref_speed_R2019a/Gearbox1/Zero inertia gear 1 ==
  theta_M : Inport
  dtheta_M : Inport  Port=2
  T_1 : Inport  Port=3
  T_loss_input : Inport  Port=4
  Add3 : Sum
  Sign & maximum for loss term : Subsystem
  theta_1 : Outport
  dtheta_1 : Outport  Port=2
  T_motor_shaft : Outport  Port=3
  wires:
  T_1/1 -> Sign & maximum for loss term/3(T_in), Add3/2
  Add3/1 -> T_motor_shaft/1
  T_loss_input/1 -> Sign & maximum for loss term/1(T_loss)
  Sign & maximum for loss term/1(T_loss_correct_sign) -> Add3/1
  dtheta_M/1 -> Sign & maximum for loss term/2(Speed), dtheta_1/1
  theta_M/1 -> theta_1/1

== system DT4V_System_Model_v17_ref_speed_R2019a/Gearbox1/Zero inertia gear 4 ==
  theta_L : Inport
  dtheta_L : Inport  Port=2
  T_4 : Inport  Port=3
  T_loss_out : Inport  Port=4
  Add3 : Sum
  Sign & maximum for loss term : Subsystem
  theta_4 : Outport
  dtheta_4 : Outport  Port=2
  T_load_shaft : Outport  Port=3
  wires:
  T_4/1 -> Sign & maximum for loss term/3(T_in), Add3/2
  Add3/1 -> T_load_shaft/1
  Sign & maximum for loss term/1(T_loss_correct_sign) -> Add3/1
  T_loss_out/1 -> Sign & maximum for loss term/1(T_loss)
  theta_L/1 -> theta_4/1
  dtheta_L/1 -> Sign & maximum for loss term/2(Speed), dtheta_4/1

== system DT4V_System_Model_v17_ref_speed_R2019a/Load Cycle/Load cycle ==
  note: M2 = load motor
  note: Speed_load is in rad/s, load model expects rpm
  Speed_load : Inport
  External load : Constant  Value=0
  Gain : Gain  Gain=30/pi
  Road slope : Constant  Value=0
  RoadLoadModel_TorqueControl : DT4V_LoadModels/RoadLoadModel_TorqueControl  Ts=Config.Ts  RL_b_ModFricSim=TP.Mdl.RL.RL_b_ModFricSim  RL_v_SmoothHoldoff_mps=TP.Mdl.RL.RL_v_SmoothHoldoff_mps  RL_a_Grav_mps2=FP.Mdl.RL.RL_ddx_Gravity_mps2  RL_Rho_Air_kgpm3=FP.Mdl.RL.RL_rho_AirDensity_kgpm3  Veh_m_Curb_kg=TP.Mdl.RL.RL_m_VehCurbWeight_kg  Veh_x_RadDyn_m=TP.Mdl.RL.RL_Rd_DynWheelRadius_m  Veh_A_Front_m2=TP.Mdl.RL.RL_A_VehFrontSurface_m2  Veh_C_Roll=TP.Mdl.RL.RL_Cr_RollCoef  Veh_C_Drag=TP.Mdl.RL.RL_Cd_AeroCoef  Veh_A0_CurbUsr_N=0  Veh_A1_CurbUsr_Nspm=0  Veh_A2_CurbUsr_Ns2pm2=0  Veh_A3_CurbUsr_Ns3pm3=0  Veh_A4_CurbUsr_Ns4pm4=0  Veh_A5_CurbUsr_Ns5pm5=0  v_BrakeBlendingSpdGrid_kph=TP.Mdl.RL.RL_v_BrakeBlendingSpdGrid_kph  r_BrakeBlendingfactor=TP.Mdl.RL.RL_r_BrakeBlendingfactor  Belt_r_TorqueRatio=FP.Belt.Belt_r_TorqueRatio
  Torque_Load : Outport
  wires:
  Gain/1 -> RoadLoadModel_TorqueControl/1
  RoadLoadModel_TorqueControl/1 -> Torque_Load/1
  External load/1 -> RoadLoadModel_TorqueControl/3
  Road slope/1 -> RoadLoadModel_TorqueControl/2
  Speed_load/1 -> Gain/1

== system DT4V_System_Model_v17_ref_speed_R2019a/Load Motor + PE/Mechanical model ==
  EM_Torque : Inport
  Load_Torque : Inport  Port=2
  Integrator2 : Integrator
  Integrator3 : Integrator
  Multiply : Gain  Gain=1/LM.J
  Sum : Sum  Inputs=|++
  "Position_Rotor " : Outport
  "Speed_Rotor " : Outport  Port=2
  wires:
  Integrator3/1 -> "Position_Rotor "/1
  Sum/1 -> Multiply/1
  Load_Torque/1 -> Sum/2
  EM_Torque/1 -> Sum/1
  Integrator2/1 -> Integrator3/1, "Speed_Rotor "/1
  Multiply/1 -> Integrator2/1

== system DT4V_System_Model_v17_ref_speed_R2019a/Load Torque/Load cycle ==
  note: M2 = load motor
  note: Speed_load is in rad/s, load model expects rpm
  Speed_load : Inport
  External load : Constant  Value=0
  Gain : Gain  Gain=30/pi
  Road slope : Constant  Value=0
  RoadLoadModel_TorqueControl : DT4V_LoadModels/RoadLoadModel_TorqueControl  Ts=Config.Ts  RL_b_ModFricSim=TP.Mdl.RL.RL_b_ModFricSim  RL_v_SmoothHoldoff_mps=TP.Mdl.RL.RL_v_SmoothHoldoff_mps  RL_a_Grav_mps2=FP.Mdl.RL.RL_ddx_Gravity_mps2  RL_Rho_Air_kgpm3=FP.Mdl.RL.RL_rho_AirDensity_kgpm3  Veh_m_Curb_kg=TP.Mdl.RL.RL_m_VehCurbWeight_kg  Veh_x_RadDyn_m=TP.Mdl.RL.RL_Rd_DynWheelRadius_m  Veh_A_Front_m2=TP.Mdl.RL.RL_A_VehFrontSurface_m2  Veh_C_Roll=TP.Mdl.RL.RL_Cr_RollCoef  Veh_C_Drag=TP.Mdl.RL.RL_Cd_AeroCoef  Veh_A0_CurbUsr_N=0  Veh_A1_CurbUsr_Nspm=0  Veh_A2_CurbUsr_Ns2pm2=0  Veh_A3_CurbUsr_Ns3pm3=0  Veh_A4_CurbUsr_Ns4pm4=0  Veh_A5_CurbUsr_Ns5pm5=0  v_BrakeBlendingSpdGrid_kph=TP.Mdl.RL.RL_v_BrakeBlendingSpdGrid_kph  r_BrakeBlendingfactor=TP.Mdl.RL.RL_r_BrakeBlendingfactor  Belt_r_TorqueRatio=FP.Belt.Belt_r_TorqueRatio
  Torque_Load : Outport
  wires:
  Gain/1 -> RoadLoadModel_TorqueControl/1
  RoadLoadModel_TorqueControl/1 -> Torque_Load/1
  External load/1 -> RoadLoadModel_TorqueControl/3
  Road slope/1 -> RoadLoadModel_TorqueControl/2
  Speed_load/1 -> Gain/1

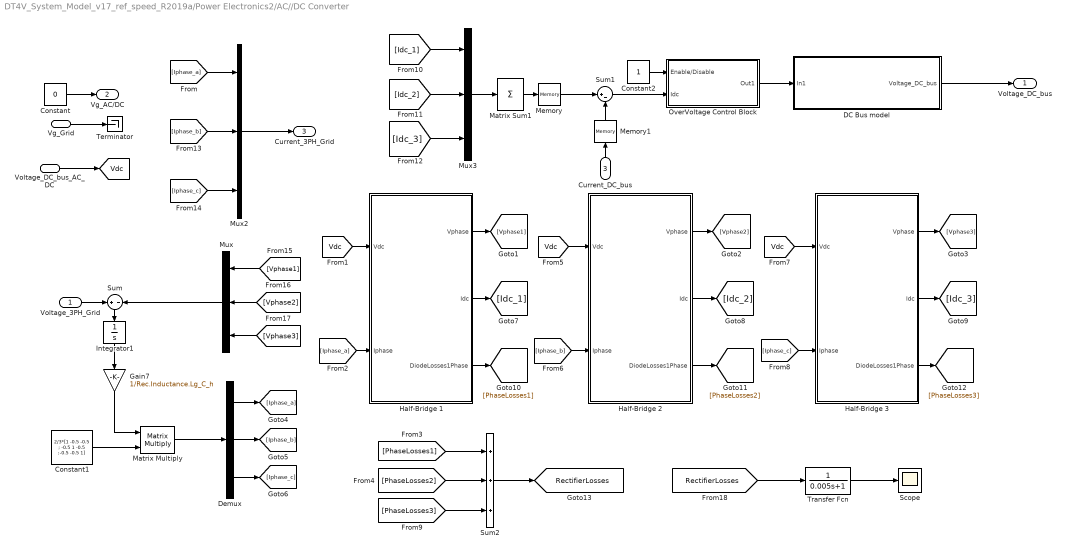
== system DT4V_System_Model_v17_ref_speed_R2019a/Power Electronics2/AC//DC Converter ==
  Voltage_3PH_Grid : Inport
  "Vg_Grid " : Inport  Port=2
  Current_DC_bus : Inport  Port=3
  Voltage_DC_bus_AC_DC : Inport  Port=4
  Constant : Constant  Value=0
  Constant1 : Constant  Value=2/3*[1 -0.5 -0.5 ; -0.5 1 -0.5 ;-0.5 -0.5 1]
  Constant2 : Constant
  DC Bus model : Subsystem
  Demux : Demux  Outputs=3
  Gain7 : Gain  Gain=1/Rec.Inductance.Lg_C_h
  "Half-Bridge 1 " : Subsystem
  Half-Bridge 2 : Subsystem
  Half-Bridge 3 : Subsystem
  Integrator1 : Integrator  IgnoreLimit=on
  Matrix Sum1 : Sum  Inputs=+
  Matrix Multiply : Product  Multiplication=Matrix(*)
  Memory : Memory  InheritSampleTime=on  LinearizeMemory=on  LinearizeAsDelay=on
  Memory1 : Memory  InheritSampleTime=on  LinearizeMemory=on  LinearizeAsDelay=on
  Mux : Mux  Inputs=3
  Mux2 : Mux  Inputs=3
  Mux3 : Mux  Inputs=3
  OverVoltage Control Block : Subsystem
  Scope : Scope
  Sum : Sum  Inputs=+-
  Sum1 : Sum  Inputs=|+-
  Sum2 : Sum  Inputs=+++
  Terminator : Terminator
  Transfer Fcn : TransferFcn  Denominator=[0.005 1]
  Voltage_DC_bus : Outport
  Vg_AC/DC : Outport  Port=2
  Current_3PH_Grid : Outport  Port=3
  tag scope: RectifierLosses=global, Vdc=global
  wires:
  [Iphase_a] -> Mux2/1
  [Iphase_c] -> Mux2/3
  [Iphase_b] -> Mux2/2
  Voltage_3PH_Grid/1 -> Sum/1
  [Idc_2] -> Mux3/2
  [Idc_1] -> Mux3/1
  [Idc_3] -> Mux3/3
  Sum1/1 -> OverVoltage Control Block/2(Idc)
  Mux3/1 -> Matrix Sum1/1
  "Vg_Grid "/1 -> Terminator/1
  Constant/1 -> Vg_AC/DC/1
  Voltage_DC_bus_AC_DC/1 -> [Vdc]
  [Vphase1] -> Mux/1
  [Vphase2] -> Mux/2
  [Vphase3] -> Mux/3
  Sum/1 -> Integrator1/1
  Constant1/1 -> Matrix Multiply/2
  Integrator1/1 -> Gain7/1
  Gain7/1 -> Matrix Multiply/1
  Demux/1 -> [Iphase_a]
  Demux/2 -> [Iphase_b]
  Demux/3 -> [Iphase_c]
  Half-Bridge 2/1(Vphase) -> [Vphase2]
  [Vdc] -> Half-Bridge 3/1(Vdc)
  [Iphase_c] -> Half-Bridge 3/2(Iphase)
  Half-Bridge 2/2(Idc) -> [Idc_2]
  Half-Bridge 3/3(DiodeLosses1Phase) -> [PhaseLosses3]
  [RectifierLosses] -> Transfer Fcn/1
  "Half-Bridge 1 "/3(DiodeLosses1Phase) -> [PhaseLosses1]
  "Half-Bridge 1 "/1(Vphase) -> [Vphase1]
  Half-Bridge 3/2(Idc) -> [Idc_3]
  "Half-Bridge 1 "/2(Idc) -> [Idc_1]
  Transfer Fcn/1 -> Scope/1
  [Iphase_b] -> Half-Bridge 2/2(Iphase)
  Sum2/1 -> [RectifierLosses]
  [PhaseLosses1] -> Sum2/1
  [Iphase_a] -> "Half-Bridge 1 "/2(Iphase)
  Half-Bridge 2/3(DiodeLosses1Phase) -> [PhaseLosses2]
  [PhaseLosses2] -> Sum2/2
  [PhaseLosses3] -> Sum2/3
  Half-Bridge 3/1(Vphase) -> [Vphase3]
  [Vdc] -> Half-Bridge 2/1(Vdc)
  [Vdc] -> "Half-Bridge 1 "/1(Vdc)
  OverVoltage Control Block/1(Out1) -> DC Bus model/1(In1)
  Constant2/1 -> OverVoltage Control Block/1(Enable/Disable)
  DC Bus model/1(Voltage_DC_bus) -> Voltage_DC_bus/1
  Mux2/1 -> Current_3PH_Grid/1
  Matrix Sum1/1 -> Memory/1
  Memory/1 -> Sum1/1
  Current_DC_bus/1 -> Memory1/1
  Memory1/1 -> Sum1/2
  Mux/1 -> Sum/2
  Matrix Multiply/1 -> Demux/1

== system DT4V_System_Model_v17_ref_speed_R2019a/Power Electronics2/DC bus  ==
  Voltage_DC_bus_AC/DC : Inport
  Vg_AC/DC : Inport  Port=2
  Current_DC_bus_DC/AC : Inport  Port=3
  Constant : Constant  Value=0
  Terminator : Terminator
  Voltage_DC_bus_DC/AC : Outport
  Vg_DC/AC : Outport  Port=2
  Current_DC_bus_AC/DC : Outport  Port=3
  wires:
  Current_DC_bus_DC/AC/1 -> Current_DC_bus_AC/DC/1
  Vg_AC/DC/1 -> Terminator/1
  Constant/1 -> Vg_DC/AC/1
  Voltage_DC_bus_AC/DC/1 -> Voltage_DC_bus_DC/AC/1

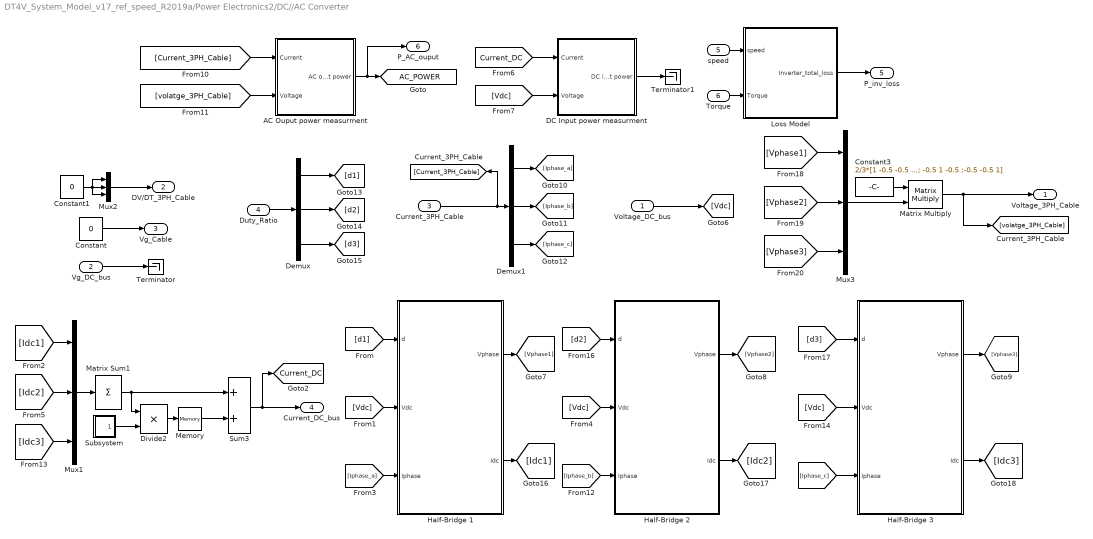
== system DT4V_System_Model_v17_ref_speed_R2019a/Power Electronics2/DC//AC Converter ==
  Voltage_DC_bus : Inport
  Vg_DC_bus : Inport  Port=2
  "Current_3PH_Cable " : Inport  Port=3
  Duty_Ratio : Inport  Port=4
  speed : Inport  Port=5
  Torque : Inport  Port=6
  AC Ouput power measurment : Subsystem
  Constant : Constant  Value=0
  Constant1 : Constant  Value=0
  Constant3 : Constant  Value=2/3*[1 -0.5 -0.5 ; -0.5 1 -0.5 ;-0.5 -0.5 1]
  DC Input power measurment : Subsystem
  Demux : Demux  Outputs=3
  Demux1 : Demux  Outputs=3
  Divide2 : Product  Inputs=**
  Half-Bridge 1 : Subsystem
  Half-Bridge 2 : Subsystem
  Half-Bridge 3 : Subsystem
  Loss Model : Subsystem
  Matrix Sum1 : Sum  Inputs=+
  Matrix Multiply : Product  Multiplication=Matrix(*)
  Memory : Memory
  Mux1 : Mux  Inputs=3
  Mux2 : Mux  Inputs=3
  Mux3 : Mux  Inputs=3
  Subsystem : Subsystem
  Sum3 : Sum
  Terminator : Terminator
  Terminator1 : Terminator
  Voltage_3PH_Cable : Outport
  DV/DT_3PH_Cable : Outport  Port=2
  "Vg_Cable " : Outport  Port=3
  Current_DC_bus : Outport  Port=4
  P_inv_loss : Outport  Port=5
  P_AC_ouput : Outport  Port=6
  tag scope: AC_POWER=global, Current_DC=global
  wires:
  Mux2/1 -> DV/DT_3PH_Cable/1
  Demux1/1 -> [Iphase_a]
  Demux1/2 -> [Iphase_b]
  Demux1/3 -> [Iphase_c]
  Duty_Ratio/1 -> Demux/1
  Demux/1 -> [d1]
  Demux/2 -> [d2]
  Demux/3 -> [d3]
  "Current_3PH_Cable "/1 -> Demux1/1, [Current_3PH_Cable]
  [Idc2] -> Mux1/2
  [Idc3] -> Mux1/3
  [Idc1] -> Mux1/1
  Mux1/1 -> Matrix Sum1/1
  Half-Bridge 1/2(Idc) -> [Idc1]
  Half-Bridge 1/1(Vphase) -> [Vphase1]
  [d1] -> Half-Bridge 1/1(d)
  Half-Bridge 3/1(Vphase) -> [Vphase3]
  Half-Bridge 2/2(Idc) -> [Idc2]
  Half-Bridge 2/1(Vphase) -> [Vphase2]
  [Iphase_a] -> Half-Bridge 1/3(Iphase)
  Half-Bridge 3/2(Idc) -> [Idc3]
  [Vdc] -> Half-Bridge 1/2(Vdc)
  [Vphase1] -> Mux3/1
  [Vphase3] -> Mux3/3
  [Vphase2] -> Mux3/2
  [d2] -> Half-Bridge 2/1(d)
  [Vdc] -> Half-Bridge 2/2(Vdc)
  [Iphase_b] -> Half-Bridge 2/3(Iphase)
  [d3] -> Half-Bridge 3/1(d)
  [Vdc] -> Half-Bridge 3/2(Vdc)
  [Iphase_c] -> Half-Bridge 3/3(Iphase)
  Vg_DC_bus/1 -> Terminator/1
  Constant/1 -> "Vg_Cable "/1
  Constant1/1 -> Mux2/3, Mux2/1, Mux2/2
  Sum3/1 -> Current_DC_bus/1, [Current_DC]
  Voltage_DC_bus/1 -> [Vdc]
  Mux3/1 -> Matrix Multiply/2
  Constant3/1 -> Matrix Multiply/1
  Matrix Multiply/1 -> Voltage_3PH_Cable/1, [volatge_3PH_Cable]
  [Current_3PH_Cable] -> AC Ouput power measurment/1(Current)
  [volatge_3PH_Cable] -> AC Ouput power measurment/2(Voltage)
  AC Ouput power measurment/1(AC ouput power) -> P_AC_ouput/1, [AC_POWER]
  [Vdc] -> DC Input power measurment/2(Voltage)
  [Current_DC] -> DC Input power measurment/1(Current)
  Matrix Sum1/1 -> Divide2/1, Sum3/1
  Loss Model/1(Inverter_total_loss) -> P_inv_loss/1
  Subsystem/1(Idc2) -> Divide2/2
  Memory/1 -> Sum3/2
  Divide2/1 -> Memory/1
  DC Input power measurment/1(DC input power) -> Terminator1/1
  Torque/1 -> Loss Model/2(Torque)
  speed/1 -> Loss Model/1(speed)

== system DT4V_System_Model_v17_ref_speed_R2019a/Voltage to Duty ratio1/Gate signal generator ==
  In1 : Inport
  Constant : Constant  Value=0.5
  Gain : Gain  Gain=1/(DCL.Cap.Vdc_C_v)
  Sum : Sum  Inputs=|++
  Out1 : Outport
  wires:
  In1/1 -> Gain/1
  Gain/1 -> Sum/1
  Constant/1 -> Sum/2
  Sum/1 -> Out1/1

== system DT4V_System_Model_v17_ref_speed_R2019a/Voltage to Duty ratio1/dqo_to_abc ==
  note: Cos(wt-2pi/3)
  note: 8
  note: Sin(wt)
  note: Sin(wt+2pi/3)
  note: 9
  note: Cos(wt+2pi/3)
  note: Sin(wt-2pi/3)
  note: 6
  note: 4
  note: Cos(wt)
  note: 7
  note: 5
  "Vdqo " : Inport
  theta : Inport  Port=2
  Constant : Constant  Value=2*pi/3
  Mux1 : Mux  Inputs=6
  Mux2 : Mux  Inputs=2
  Mux3 : Mux  Inputs=3
  Sum : Sum  Inputs=+-
  Sum1 : Sum
  Trigonometric Function : Trigonometry
  Trigonometric Function1 : Trigonometry  Operator=cos
  Trigonometric Function2 : Trigonometry
  Trigonometric Function3 : Trigonometry  Operator=cos
  Trigonometric Function4 : Trigonometry
  Trigonometric Function5 : Trigonometry  Operator=cos
  a : Fcn  Expr=-u(2)*u(4)+u(1)*u(5)+u(3)
  b : Fcn  Expr=-u(2)*u(6)+u(1)*u(7)+u(3)
  c : Fcn  Expr=-u(2)*u(8)+u(1)*u(9)+u(3)
  abc : Outport
  wires:
  c/1 -> Mux3/3
  Trigonometric Function/1 -> Mux1/1
  Sum1/1 -> Trigonometric Function5/1, Trigonometric Function4/1
  Sum/1 -> Trigonometric Function3/1, Trigonometric Function2/1
  theta/1 -> Trigonometric Function/1, Trigonometric Function1/1, Sum1/1, Sum/1
  Constant/1 -> Sum1/2, Sum/2
  b/1 -> Mux3/2
  Trigonometric Function1/1 -> Mux1/2
  "Vdqo "/1 -> Mux2/1
  Trigonometric Function5/1 -> Mux1/6
  Trigonometric Function4/1 -> Mux1/5
  Trigonometric Function3/1 -> Mux1/4
  Mux1/1 -> Mux2/2
  Mux3/1 -> abc/1
  Trigonometric Function2/1 -> Mux1/3
  Mux2/1 -> b/1, a/1, c/1
  a/1 -> Mux3/1

== system DT4V_System_Model_v17_ref_speed_R2019a/Drive Motor/Electromagnetic Model/DQ-transform  ==
  note: v_d
  note: v_q
  note: v_beta
  note: v_alpha
  note: theta_el
  Voltage_3PH : Inport
  Rotor_position : Inport  Port=2
  Constant : Constant  Value=EM.Np
  Demux : Demux  Outputs=2
      settings: DisplayOption=none
  Product{,1,3..4,7} (5 alike) : Product  InputSameDT=on  SaturateOnIntegerOverflow=on  OutDataTypeStr=Inherit: Same as first input
  Sum1 : Sum  Inputs=|++  InputSameDT=on  SaturateOnIntegerOverflow=on  OutDataTypeStr=Inherit: Same as first input
  Sum4 : Sum  Inputs=|+-  InputSameDT=on  SaturateOnIntegerOverflow=on  OutDataTypeStr=Inherit: Same as first input
  Tclark : Gain  Gain=EM.TaA  Multiplication=Matrix(K*u)  SaturateOnIntegerOverflow=on  OutDataTypeStr=Inherit: Same as input  ParamDataTypeStr=Inherit: Same as input
  Trigonometric Function2 : Trigonometry  Operator=cos
  Trigonometric Function3 : Trigonometry
  V_q : Outport
  "V_d " : Outport  Port=2
  wires:
  Trigonometric Function3/1 -> Product4/2, Product7/2
  Product1/1 -> Sum1/1
  Constant/1 -> Product/2
  Product3/1 -> Sum4/1
  Product/1 -> Trigonometric Function2/1, Trigonometric Function3/1
  Demux/1 -> Product1/1, Product7/1
  Tclark/1 -> Demux/1
  Demux/2 -> Product3/1, Product4/1
  Product4/1 -> Sum1/2
  Trigonometric Function2/1 -> Product1/2, Product3/2
  Product7/1 -> Sum4/2
  Voltage_3PH/1 -> Tclark/1
  Sum1/1 -> V_q/1
  Rotor_position/1 -> Product/1
  Sum4/1 -> "V_d "/1

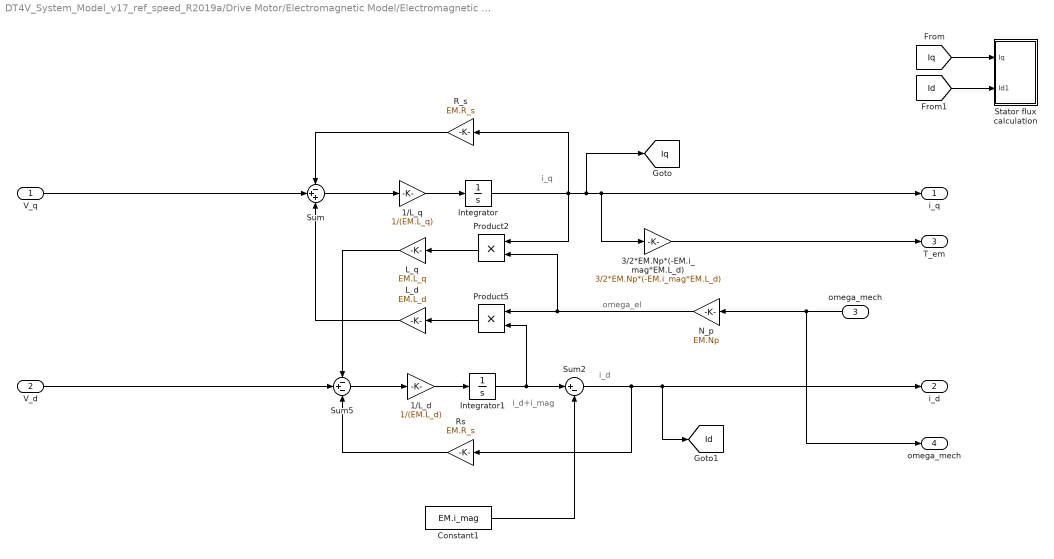
== system DT4V_System_Model_v17_ref_speed_R2019a/Drive Motor/Electromagnetic Model/Electromagnetic model ==
  note: i_d+i_mag
  note: omega_el
  note: i_d
  note: i_q
  "V_q " : Inport
  "V_d " : Inport  Port=2
  "omega_mech " : Inport  Port=3
  1/L_d : Gain  Gain=1/(EM.L_d)
  1/L_q : Gain  Gain=1/(EM.L_q)
  3/2*EM.Np*(-EM.i_mag*EM.L_d) : Gain  Gain=3/2*EM.Np*(-EM.i_mag*EM.L_d)
  Constant1 : Constant  Value=EM.i_mag
  Integrator : Integrator  UpperSaturationLimit=38  LowerSaturationLimit=-38
  Integrator1 : Integrator  InitialCondition=EM.i_mag
  L_d : Gain  Gain=EM.L_d
  L_q : Gain  Gain=EM.L_q
  N_p : Gain  Gain=EM.Np
  Product2 : Product  RndMeth=Zero
  Product5 : Product  RndMeth=Zero
  R_s : Gain  Gain=EM.R_s
  Rs : Gain  Gain=EM.R_s
  Stator flux calculation : Subsystem
  Sum : Sum  Inputs=-++
  Sum2 : Sum  Inputs=|+-
  Sum5 : Sum  Inputs=-+-
  "i_q " : Outport
  "i_d " : Outport  Port=2
  "T_em " : Outport  Port=3
  omega_mech : Outport  Port=4
  tag scope: Id=global, Iq=global
  wires:
  Sum5/1 -> 1/L_d/1
  Product5/1 -> L_d/1
  L_q/1 -> Sum5/1
  "V_d "/1 -> Sum5/2
  Sum2/1 -> Rs/1, "i_d "/1, [Id]
  R_s/1 -> Sum/1
  Integrator1/1 -> Sum2/1, Product5/2
  1/L_d/1 -> Integrator1/1
  Sum/1 -> 1/L_q/1
  Rs/1 -> Sum5/3
  "omega_mech "/1 -> omega_mech/1, N_p/1
  Product2/1 -> L_q/1
  N_p/1 -> Product5/1, Product2/2
  L_d/1 -> Sum/3
  Constant1/1 -> Sum2/2
  "V_q "/1 -> Sum/2
  3/2*EM.Np*(-EM.i_mag*EM.L_d)/1 -> "T_em "/1
  [Iq] -> Stator flux calculation/1("Iq ")
  [Id] -> Stator flux calculation/2(Id1)
  1/L_q/1 -> Integrator/1
  Integrator/1 -> Product2/1, R_s/1, 3/2*EM.Np*(-EM.i_mag*EM.L_d)/1, "i_q "/1, [Iq]

== system DT4V_System_Model_v17_ref_speed_R2019a/Drive Motor/Electromagnetic Model/Inverse DQ-transform ==
  note: i_beta
  note: i_alpha
  note: theta_el
  i_q : Inport
  i_d : Inport  Port=2
  Rotor_position : Inport  Port=3
  Mux1 : Mux  Inputs=2
  Np : Constant  Value=EM.Np
  Product{6,8..11} (5 alike) : Product  InputSameDT=on  SaturateOnIntegerOverflow=on  OutDataTypeStr=Inherit: Same as first input
  Sum6 : Sum  Inputs=|+-  InputSameDT=on  SaturateOnIntegerOverflow=on  OutDataTypeStr=Inherit: Same as first input
  Sum7 : Sum  Inputs=|++  InputSameDT=on  SaturateOnIntegerOverflow=on  OutDataTypeStr=Inherit: Same as first input
  Tclark invers : Gain  Gain=EM.TAa  Multiplication=Matrix(K*u)  SaturateOnIntegerOverflow=on  OutDataTypeStr=Inherit: Same as input  ParamDataTypeStr=Inherit: Same as input
  Trigonometric Function1 : Trigonometry  Operator=cos
  Trigonometric Function4 : Trigonometry
  Current_3PH : Outport
  wires:
  Product9/1 -> Sum7/1
  Mux1/1 -> Tclark invers/1
  Trigonometric Function1/1 -> Product6/2, Product9/2
  Sum6/1 -> Mux1/1
  Product8/1 -> Trigonometric Function1/1, Trigonometric Function4/1
  Np/1 -> Product8/2
  Tclark invers/1 -> Current_3PH/1
  Product10/1 -> Sum6/2
  Trigonometric Function4/1 -> Product10/2, Product11/2
  Rotor_position/1 -> Product8/1
  i_q/1 -> Product11/1, Product6/1
  Sum7/1 -> Mux1/2
  Product6/1 -> Sum6/1
  Product11/1 -> Sum7/2
  i_d/1 -> Product10/1, Product9/1
